simulink model "my_sim_master"  (R2020a)
settings: Solver=ode45  StartTime=0.0  StopTime=2  FixedStep=0.001  RelTol=1e-3  EnableMultiTasking=on
settings Model: ExtModeTrigMode=oneshot  ExtModeArmWhenConnect=off  Creator=td  LastModifiedBy=td
settings DataIOCC: SaveFormat=Array  SignalLoggingSaveFormat=ModelDataLogs  ReturnWorkspaceOutputs=off  SignalLoggingName=sigsOut
settings OptimizationCC: BooleanDataType=off
settings DebuggingCC: SaveWithParameterizedLinksMsg=none  UnderspecifiedInitializationDetection=Classic  MergeDetectMultiDrivingBlocksExec=none  SignalResolutionControl=TryResolveAllWithWarning  MultiTaskDSMMsg=warning  MultiTaskCondExecSysMsg=none
settings HardwareCC: ProdBitPerPointer=32  ProdBitPerSizeT=32  ProdBitPerPtrDiffT=32  ProdLargestAtomicFloat=None  ProdIntDivRoundTo=Undefined  ProdEndianess=Unspecified  ProdWordSize=32  ProdHWDeviceType=32-bit Generic  TargetUnknown=on
settings ModelReferenceCC: PropagateSignalLabelsOutOfModel=off
settings GRTTargetCC: CombineOutputUpdateFcns=off  GRTInterface=on
settings ConfigComp: CovMetricSettings=dw  CovHtmlReporting=on  CovSaveCumulativeToWorkspaceVar=on  CovSaveSingleToWorkspaceVar=on

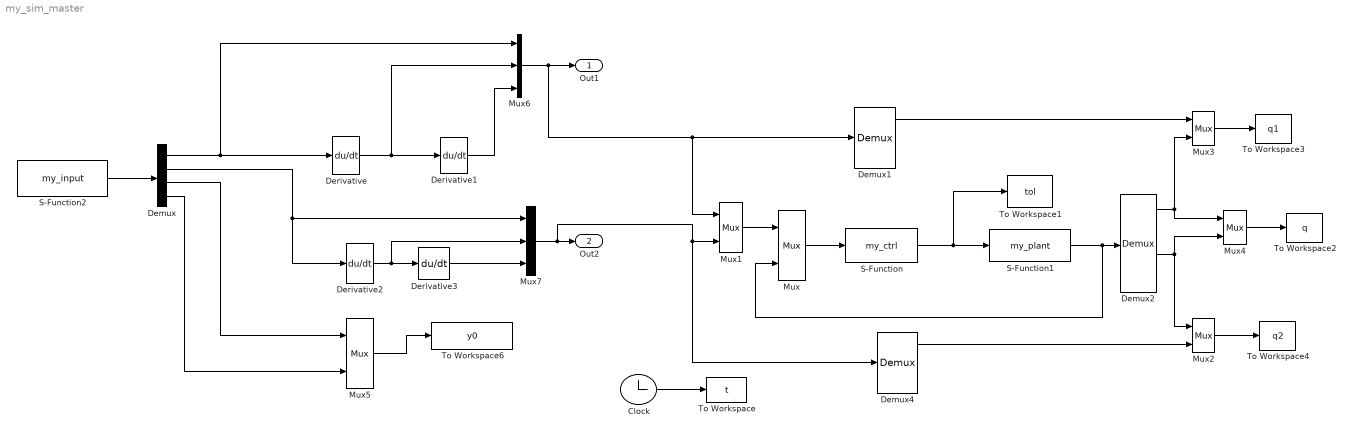
== system my_sim_master ==
  Clock : Clock
  Demux : Demux
      settings: DisplayOption=none
  Demux1 : Demux  Outputs=3
      settings: DisplayOption=none
  Demux2 : Demux
      settings: DisplayOption=none
  Demux4 : Demux  Outputs=3
      settings: DisplayOption=none
  Derivative{,1..3} (4 alike) : Derivative
  Mux{,1..5} (6 alike) : Mux  Inputs=2
  Mux6 : Mux  Inputs=3
  Mux7 : Mux  Inputs=3
  S-Function : S-Function  FunctionName=my_ctrl  SFunctionDeploymentMode=off  EnableBusSupport=off
  S-Function1 : S-Function  FunctionName=my_plant  Parameters=0.1,0.1  SFunctionDeploymentMode=off  EnableBusSupport=off
  S-Function2 : S-Function  FunctionName=my_input  SFunctionDeploymentMode=off  EnableBusSupport=off
  To Workspace : ToWorkspace  VariableName=t  SampleTime=-1
  To Workspace1 : ToWorkspace  VariableName=tol  SampleTime=-1
  To Workspace2 : ToWorkspace  VariableName=q  SampleTime=-1
  To Workspace3 : ToWorkspace  VariableName=q1  SampleTime=-1
  To Workspace4 : ToWorkspace  VariableName=q2  SampleTime=-1
  To Workspace6 : ToWorkspace  VariableName=y0  SampleTime=-1
  Out1 : Outport
  Out2 : Outport  Port=2
  wires:
  Mux/1 -> S-Function/1
  Mux2/1 -> To Workspace4/1
  Mux3/1 -> To Workspace3/1
  S-Function/1 -> S-Function1/1, To Workspace1/1
  S-Function1/1 -> Mux/2, Demux2/1
  Demux2/3 -> Mux2/1, Mux4/2
  Mux1/1 -> Mux/1
  Demux4/1 -> Mux2/2
  Mux6/1 -> Mux1/1, Demux1/1, Out1/1
  Mux7/1 -> Mux1/2, Demux4/1, Out2/1
  Demux2/1 -> Mux3/2, Mux4/1
  Demux1/1 -> Mux3/1
  Clock/1 -> To Workspace/1
  Mux4/1 -> To Workspace2/1
  Mux5/1 -> To Workspace6/1
  Derivative2/1 -> Derivative3/1, Mux7/2
  Demux/2 -> Derivative2/1, Mux7/1
  Derivative/1 -> Derivative1/1, Mux6/2
  Derivative3/1 -> Mux7/3
  Demux/1 -> Derivative/1, Mux6/1
  Demux/3 -> Mux5/1
  Derivative1/1 -> Mux6/3
  Demux/4 -> Mux5/2
  S-Function2/1 -> Demux/1
